simulink model "LSM_4p6U10_v01_06022022_NEW_ECC_2019a"  (R2019a)
settings: Solver=FixedStepAuto  StartTime=0.0  StopTime=Inf  FixedStep=Ts_lowspeed  RelTol=1e-3  EnableMultiTasking=on
PostLoadFcn:
  | , if any(exist('dsrtsu_mdlpostloadfcn', 'file') == [2, 3, 6]), try dsrtsu_mdlpostloadfcn('Execute', bdroot); catch fprintf('Error in PostLoadFcn (dsrtsu_mdlpostloadfcn) for model "%s":\n %s\n', bdroot, lasterr); end, end,
values from neighbouring files (symbols this model uses):
  Ts_lowspeed = 0.05    [Parameters_4p6U10.m]
undefined symbols (not defined in the file or in its folder): Down, GPTRIP1SEL, GPTRIP2SEL, TZ1, TZ2, Up
libraries: simulink x91, simulink_extras x25, c2802xlib x12, c2837xDlib x8, c280xlib x8
(part 1 of 2)
PreSaveFcn:
  | , if any(exist('dsmpb_private', 'file') == [2, 3, 6]), try, dsmpb_private('dsmpb_mdlclblib', 'PreSave', bdroot); catch, disp(lasterr); end, end,
CloseFcn:
  | , if any(exist('dsmpb_private', 'file') == [2, 3, 6]), try, dsmpb_private('dsmpb_mdlclblib', 'Close', bdroot); catch, disp(lasterr); end, end,
settings Model: DSRTSU_INTERNAL_RTI_VER=500  DSRTSU_INTERNAL_RTI_TYPE=rti1007  DSRTSU_INTERNAL_RTIFPGA=90  DSMPB_DATASERVER_ModelPortLibVersion1=8  DSMPB_DATASERVER_DataServerVersion1=6  DSMPB_DATASERVER_DataServerStreamVersion1=3  SimulationMode=external  ExtModeTrigDuration=8  Creator=Christos  LastModifiedBy=ThermoLift
settings DataIOCC: ReturnWorkspaceOutputs=off
settings OptimizationCC: BlockReduction=off  ConditionallyExecuteInputs=off  DefaultUnderspecifiedDataType=single  EnhancedBackFolding=on  PassReuseOutputArgsAs=Individual arguments  MaxStackSize=512  OptimizeBlockOrder=speed
settings DebuggingCC: AlgebraicLoopMsg=none  ArtificialAlgebraicLoopMsg=none  ParameterPrecisionLossMsg=none  ParameterTunabilityLossMsg=error  SFUnexpectedBacktrackingDiag=warning  SFNoUnconditionalDefaultTransitionDiag=warning  SFExecutionAtInitializationDiag=none  ArithmeticOperatorsInVariantConditions=warning
settings HardwareCC: ProdBitPerChar=16  ProdBitPerInt=16  ProdBitPerPointer=32  ProdBitPerSizeT=32  ProdBitPerPtrDiffT=32  ProdLargestAtomicInteger=Integer  ProdLargestAtomicFloat=None  ProdWordSize=16  ProdLongLongMode=on  ProdHWDeviceType=Texas Instruments->C2000  TargetIntDivRoundTo=Zero  TargetEndianess=BigEndian  TargetHWDeviceType=Custom Processor->Custom
settings SFSimCC: SimUseLocalCustomCode=off  MATLABDynamicMemAlloc=off
settings RTWCC: SystemTargetFile=ert.tlc  HardwareBoard=TI Delfino F28379D LaunchPad  TLCOptions=-aInlineSetEventsForThisBaseRateFcn=TLC_FALSE -aSuppressMultiTaskScheduler=TLC_FALSE -aRateBasedStepFcn=1  TemplateMakefile=ert_default_tmf  GenerateReport=on  RTWUseLocalCustomCode=off  RTWUseSimCustomCode=on  Toolchain=Texas Instruments Code Composer Studio (C2000)  IncludeHyperlinkInReport=on  LaunchReport=on  GenerateTraceInfo=on  GenerateTraceReport=on  GenerateTraceReportSl=on  GenerateTraceReportSf=on  GenerateTraceReportEml=on
settings CodeAppCC: ForceParamTrailComments=on  IgnoreCustomStorageClasses=off  OperatorAnnotations=on  SimulinkDataObjDesc=on  SFDataObjDesc=on  InsertBlockDesc=on  StateflowObjectComments=on
settings ERTTargetCC: CodeReplacementLibrary=TI C28x  SupportContinuousTime=on
settings ConfigComp: CovMetricSettings=dw  CovSaveCumulativeToWorkspaceVar=on  CovSaveSingleToWorkspaceVar=on  CovExternalEMLEnable=off
settings SimscapeCC: SimscapeNormalizeSystem=off

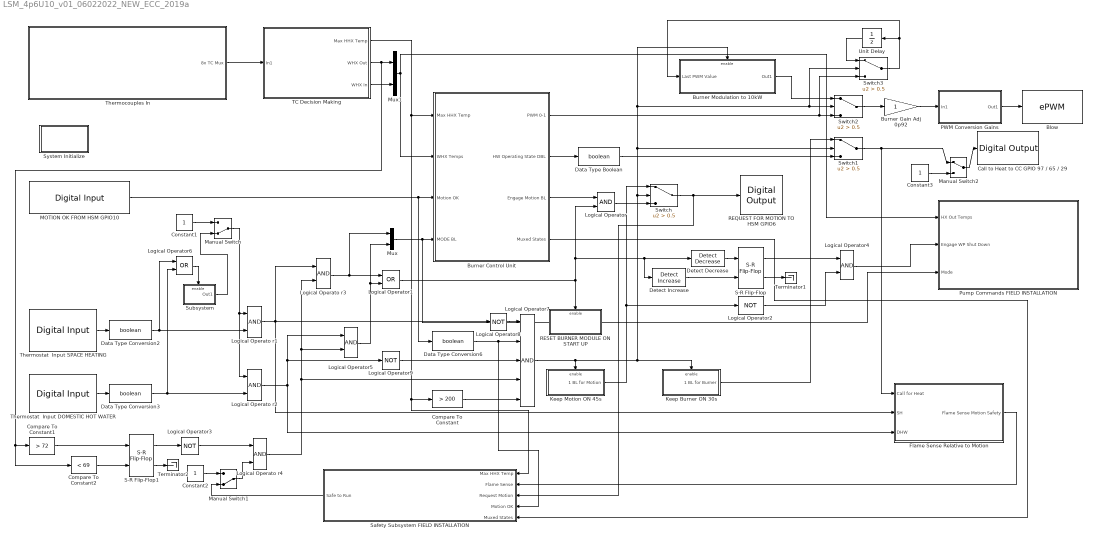
== system LSM_4p6U10_v01_06022022_NEW_ECC_2019a ==
  Blow : c2802xlib/ePWM  useModule=ePWM3  ePWMxLINKTBPRD=Not Linked  periodUnits=Clock cycles  timerSource=Specify via dialog  timerPeriod_clk=16000  timerPeriod_sec=0.0001  tbshadow=Counter equals to zero  countingMode=Up-Down  phaseActiveEnable=Disable  phaseDirection=Count down after sync  phaseActive=0  synchronizationEnable=off  dcaevt1Sync=off  dcbevt1Sync=off  synchronizationOption=Disable  clockPrescale=1  HSclockPrescale=1  enswap=off  ePWMxAStatus=off  ePWMxAactionLogic1=Set  ePWMxAactionLogic2=Clear  ePWMxAactionLogic3=Clear  ePWMxAactionLogic4=Set  ePWMxAactionLogic5=Do nothing  ePWMxAactionLogic6=Do nothing  ePWMxALoadMode=Load on counter equals to zero (CTR=Zero)  ePWMxACSFenable=off  ePWMxACSFvalue=Forcing disable  ePWMxASFreload=Zero  ePWMxBStatus=on  ePWMxBactionLogic1=Set  ePWMxBactionLogic2=Clear  ePWMxBactionLogic3=Clear  ePWMxBactionLogic4=Set  ePWMxBactionLogic5=Do nothing  ePWMxBactionLogic6=Do nothing  ePWMxBLoadMode=Load on counter equals to zero (CTR=Zero)  ePWMxBCSFenable=off  ePWMxBCSFvalue=Forcing disable  ePWMxBSFreload=Zero  ePWNxBOutWay=off  ePWMxLINKCMPA=Not Linked  CMPAUnits=Clock cycles  CMPASource=Input port  CMPAValue_per=0  CMPAValue_clk=32000  enCMPAshadow=Counter equals to zero  ePWMxLINKCMPB=Not Linked  CMPBUnits=Clock cycles  CMPBSource=Specify via dialog  CMPBValue_per=50  CMPBValue_clk=32000  enCMPBshadow=Counter equals to zero  ePWMxLINKCMPC=Not Linked  CMPCUnits=Clock cycles  CMPCSource=Specify via dialog  CMPCValue_per=50  CMPCValue_clk=032000  enCMPCshadow=Counter equals to zero  ePWMxLINKCMPD=Not Linked  CMPDUnits=Clock cycles  CMPDSource=Specify via dialog  CMPDValue_per=50  CMPDValue_clk=32000  enCMPDshadow=Counter equals to zero  enableDBePWMxA=off  enableDBePWMxB=off  enhalfcycle=off  DBpolarity=Active high (AH)  DBedgeDelay=Positive  DBSource_ePWMxA=ePWMxA  DBSource_ePWMxB=ePWMxA  DBperiodSource=Specify via dialog  REDperiod=0  FEDperiod=0  adcstartModuleA=off  adcrequestEventA=First event  adcstartEventA=Digital Compare Module A Event 1 start of conversion (DCAEVT1.soc)  adcstartEventA_type2=Digital Compare Module A Event 1 start of conversion (DCAEVT1.soc)  adcstartModuleB=off  adcrequestEventB=First event  adcstartEventB=Counter equals to zero (CTR=Zero)  adcstartEventB_type2=Counter equals to zero (CTR=Zero)  intEn=off  intPrd=First event  intSel=Counter equals to zero (CTR=Zero)  intSel_type2=Counter equals to zero (CTR=Zero)  hrpe=off  enHRPWM=off  HRPWM_LoadMode=Counter equals to period (CTR=PRD)  HRPWM_CTLMode=Duty or Period control mode  HRPWM_EDGMode=Both edge  hrpeb=off  enHRPWMB=off  HRPWM_LoadModeB=Counter equals to zero (CTR=ZERO)  HRPWM_CTLModeB=Duty or Period control mode  HRPWM_EDGModeB=Both edge  enSFO=on  enautoconv=on  chopperEnable=off  chopperFrequency=1  chopperFirstwidth=1  chopperDuty=12.5%  tripZonesource=Specify via dialog  tzselOSHT1=off  tzselOSHT2=off  tzselOSHT3=off  tzselOSHDCAEV1=off  tzselOSHDCBEV1=off  tzselCBC1=off  tzselCBC2=off  tzselCBC3=off  tzselCBCDCAEV2=off  tzselCBCDCBEV2=off  tzselOSHT4=off  tzselOSHT5=off  tzselOSHT6=off  tzselCBC4=off  tzselCBC5=off  tzselCBC6=off  enTzOstIntr=off  enTzCbcIntr=off  enTzDCAEVT1Intr=off  enTzDCAEVT2Intr=off  enTzDCBEVT1Intr=off  enTzDCBEVT2Intr=off  ePWMxAforced=No action  ePWMxBforced=No action  DCAEVT1forced=No action  DCBEVT1forced=No action  DCAEVT2forced=No action  DCBEVT2forced=No action  dcah=Trip Zone 1 input (TZ1)  dcal=Trip Zone 2 input (TZ2)  dcbh=Trip Zone 1 input (TZ1)  dcbl=Trip Zone 2 input (TZ2)  dcah_type2=GPTRIP1SEL/(TZ1)  dcal_type2=GPTRIP2SEL/(TZ2)  dcbh_type2=GPTRIP1SEL/(TZ1)  dcbl_type2=GPTRIP2SEL/(TZ2)  gendcaevt1=Event disabled  gendcaevt2=Event disabled  gendcbevt1=Event disabled  gendcbevt2=Event disabled  dcaevt1src=DCAEVT1 with sync  dcaevt2src=DCAEVT2 with sync  dcbevt1src=DCBEVT1 with sync  dcbevt2src=DCBEVT2 with sync  pulsesel=Counter equals to zero (CTR=Zero)  blankinv=off  blankoffset=0  blankwidth=0  evsrcsel=Filtered version of DCAEVT1 (DCAEVT1FILT)  encape=off  PwmType=C2000_Type4
  Burner Gain Adj 0p92 : Gain
  Burner Control Unit : Subsystem
  Burner Modulation to 10kW : Subsystem
  Call to Heat to CC GPIO 97 / 65 / 29 : c2837xDlib/Digital Output  GPIO_Number=GPIO0~GPIO7  GPIO_Bit0=off  GPIO_BIT0_Toggle=off  GPIO_Bit1=off  GPIO_BIT1_Toggle=off  GPIO_Bit2=off  GPIO_BIT2_Toggle=off  GPIO_Bit3=on  GPIO_BIT3_Toggle=off  GPIO_Bit4=off  GPIO_BIT4_Toggle=off  GPIO_Bit5=off  GPIO_BIT5_Toggle=off  GPIO_Bit6=off  GPIO_BIT6_Toggle=off  GPIO_Bit7=off  GPIO_BIT7_Toggle=off
      settings: SourceProductBaseCode=TIC2000
  Compare To Constant : simulink/Logic and Bit Operations/Compare To Constant  relop=>  const=200  OutDataTypeStr=boolean
  Compare To Constant1 : simulink/Logic and Bit Operations/Compare To Constant  relop=>  const=72  OutDataTypeStr=boolean
  Compare To Constant2 : simulink/Logic and Bit Operations/Compare To Constant  relop=<  const=69  OutDataTypeStr=boolean
  Constant1 : Constant  OutDataTypeStr=boolean
  Constant2 : Constant  OutDataTypeStr=boolean
  Constant3 : Constant  OutDataTypeStr=boolean
  Data Type Boolean : DataTypeConversion  OutDataTypeStr=boolean
  Data Type Conversion2 : DataTypeConversion  OutDataTypeStr=boolean
  Data Type Conversion3 : DataTypeConversion  OutDataTypeStr=boolean
  Data Type Conversion6 : DataTypeConversion  OutDataTypeStr=boolean
  Detect Decrease : simulink/Logic and Bit Operations/Detect Decrease  vinit=0.0  OutDataTypeStr=boolean
  Detect Increase : simulink/Logic and Bit Operations/Detect Increase  vinit=0.0  OutDataTypeStr=boolean
  Flame Sense Relative to Motion : Subsystem
  Keep Burner ON 30s : Subsystem
  Keep Motion ON 45s : Subsystem
  Logical Operato r{1..4} (4 alike) : Logic  AllPortsSameDT=off  OutDataTypeStr=boolean
  Logical Operator : Logic  AllPortsSameDT=off  OutDataTypeStr=boolean
  Logical Operator1 : Logic  Operator=OR  AllPortsSameDT=off  OutDataTypeStr=boolean
  Logical Operator{2..3,8..9} (4 alike) : Logic  Operator=NOT  AllPortsSameDT=off  OutDataTypeStr=boolean
  Logical Operator4 : Logic  AllPortsSameDT=off  OutDataTypeStr=boolean
  Logical Operator5 : Logic  AllPortsSameDT=off  OutDataTypeStr=boolean
  Logical Operator6 : Logic  Operator=OR  AllPortsSameDT=off  OutDataTypeStr=boolean
  Logical Operator7 : Logic  Inputs=5  AllPortsSameDT=off  OutDataTypeStr=boolean
  MOTION OK FROM HSM GPIO10 : c2837xDlib/Digital Input  GPIO_Number=GPIO8~GPIO15  GPIO_Bit0=off  GPIO_Bit1=off  GPIO_Bit2=on  GPIO_Bit3=off  GPIO_Bit4=off  GPIO_Bit5=off  GPIO_Bit6=off  GPIO_Bit7=off  sampleTime=Ts_lowspeed  dataType=boolean  GPIO_Bit0_Qualification=Sync to SYSCLKOUT  GPIO_Bit1_Qualification=Sync to SYSCLKOUT  GPIO_Bit2_Qualification=Sync to SYSCLKOUT  GPIO_Bit3_Qualification=Sync to SYSCLKOUT  GPIO_Bit4_Qualification=Sync to SYSCLKOUT  GPIO_Bit5_Qualification=Sync to SYSCLKOUT  GPIO_Bit6_Qualification=Sync to SYSCLKOUT  GPIO_Bit7_Qualification=Sync to SYSCLKOUT  Qualification_Period=-1
      settings: SourceProductBaseCode=TIC2000
  Manual Switch : ManualSwitch  CurrentSetting=0
  Manual Switch1 : ManualSwitch  CurrentSetting=0
  Manual Switch2 : ManualSwitch
  Mux : Mux  Inputs=2
  Mux1 : Mux  Inputs=2
  PWM Conversion Gains : Subsystem
  Pump Commands FIELD INSTALLATION : Subsystem
  REQUEST FOR MOTION TO HSM GPIO6 : c2837xDlib/Digital Output  GPIO_Number=GPIO0~GPIO7  GPIO_Bit0=off  GPIO_BIT0_Toggle=off  GPIO_Bit1=off  GPIO_BIT1_Toggle=off  GPIO_Bit2=off  GPIO_BIT2_Toggle=off  GPIO_Bit3=off  GPIO_BIT3_Toggle=off  GPIO_Bit4=off  GPIO_BIT4_Toggle=off  GPIO_Bit5=off  GPIO_BIT5_Toggle=off  GPIO_Bit6=on  GPIO_BIT6_Toggle=off  GPIO_Bit7=off  GPIO_BIT7_Toggle=off
      settings: SourceProductBaseCode=TIC2000
  RESET BURNER MODULE ON START UP : Subsystem
  S-R Flip-Flop : simulink_extras/Flip Flops/S-R Flip-Flop  initial_condition=0
  S-R Flip-Flop1 : simulink_extras/Flip Flops/S-R Flip-Flop  initial_condition=0
  Safety Subsystem FIELD INSTALLATION : Subsystem
  Subsystem : Subsystem
  Switch{,1..3} (4 alike) : Switch  Criteria=u2 > Threshold  Threshold=0.5
  System Initialize : Subsystem  mask(System Initialize){ShowInLibBrowser=0}
      mask prompts: ShowInLibBrowser "Simulink:masks:CustCodeMaskParam1_MP"
      settings: CopyFcn=cccopyfcn(gcb)  OpenFcn=ccopenfcn('System Initialize Function')
      mask Help: eval('feval(''rtwprivate'',''rtwhelpview'',''rtw_sys_initialize_block'')');
      mask Display: disp('System\nInitialize');
  TC Decision Making : Subsystem
  Terminator1 : Terminator
  Terminator2 : Terminator
  Thermocouples In : Subsystem
  Thermostat  Input DOMESTIC HOT WATER : c2837xDlib/Digital Input  GPIO_Number=GPIO16~GPIO23  GPIO_Bit0=off  GPIO_Bit1=off  GPIO_Bit2=on  GPIO_Bit3=off  GPIO_Bit4=off  GPIO_Bit5=off  GPIO_Bit6=off  GPIO_Bit7=off  sampleTime=Ts_lowspeed  dataType=boolean  GPIO_Bit0_Qualification=Sync to SYSCLKOUT  GPIO_Bit1_Qualification=Sync to SYSCLKOUT  GPIO_Bit2_Qualification=Sync to SYSCLKOUT  GPIO_Bit3_Qualification=Sync to SYSCLKOUT  GPIO_Bit4_Qualification=Sync to SYSCLKOUT  GPIO_Bit5_Qualification=Sync to SYSCLKOUT  GPIO_Bit6_Qualification=Sync to SYSCLKOUT  GPIO_Bit7_Qualification=Sync to SYSCLKOUT  Qualification_Period=-1
      settings: SourceProductBaseCode=TIC2000
  Thermostat  Input SPACE HEATING : c2837xDlib/Digital Input  GPIO_Number=GPIO32~GPIO39  GPIO_Bit0=on  GPIO_Bit1=off  GPIO_Bit2=off  GPIO_Bit3=off  GPIO_Bit4=off  GPIO_Bit5=off  GPIO_Bit6=off  GPIO_Bit7=off  sampleTime=Ts_lowspeed  dataType=boolean  GPIO_Bit0_Qualification=Sync to SYSCLKOUT  GPIO_Bit1_Qualification=Sync to SYSCLKOUT  GPIO_Bit2_Qualification=Sync to SYSCLKOUT  GPIO_Bit3_Qualification=Sync to SYSCLKOUT  GPIO_Bit4_Qualification=Sync to SYSCLKOUT  GPIO_Bit5_Qualification=Sync to SYSCLKOUT  GPIO_Bit6_Qualification=Sync to SYSCLKOUT  GPIO_Bit7_Qualification=Sync to SYSCLKOUT  Qualification_Period=-1
      settings: SourceProductBaseCode=TIC2000
  Unit Delay : UnitDelay  SampleTime=-1  HasFrameUpgradeWarning=on
  wires:
  Logical Operator/1 -> Switch/3
  Mux/1 -> Pump Commands FIELD INSTALLATION/3(Mode), Burner Control Unit/4(MODE BL)
  MOTION OK FROM HSM GPIO10/1 -> Burner Control Unit/3(Motion OK), Data Type Conversion6/1
  Logical Operato r2/1 -> Flame Sense Relative to Motion/3(DHW), Logical Operator5/1, Logical Operator9/1
  Logical Operato r1/1 -> Flame Sense Relative to Motion/2(SH), Logical Operator8/1, Logical Operato r3/1
  Thermostat  Input SPACE HEATING/1 -> Data Type Conversion2/1
  Burner Control Unit/3(Engage Motion BL) -> Logical Operator/1
  Thermostat  Input DOMESTIC HOT WATER/1 -> Data Type Conversion3/1
  Data Type Boolean/1 -> Switch1/3
  Logical Operato r3/1 -> Mux/1, Logical Operator1/1
  Logical Operator1/1 -> RESET BURNER MODULE ON START UP/Enable, Logical Operator/2, Detect Increase/1, Detect Decrease/1
  Logical Operator5/1 -> Mux/2, Logical Operator1/2
  Burner Control Unit/2(HW Operating State DBL) -> Data Type Boolean/1
  Data Type Conversion6/1 -> Safety Subsystem FIELD INSTALLATION/4(Motion OK), Logical Operator7/2
  Logical Operator8/1 -> Logical Operator7/1
  Logical Operator9/1 -> Logical Operator7/3
  Logical Operator7/1 -> Burner Modulation to 10kW/Enable, Switch3/2, Switch2/2, Switch1/2, Switch/2, Keep Burner ON 30s/Enable, Keep Motion ON 45s/Enable
  Keep Motion ON 45s/1(1 BL for Motion) -> Logical Operator2/1, Switch/1
  Keep Burner ON 30s/1(1 BL for Burner) -> Switch1/1
  Switch1/1 -> Flame Sense Relative to Motion/1(Call for Heat), Manual Switch2/1
  Logical Operato r4/1 -> Logical Operato r3/2, Logical Operator5/2, Logical Operator7/4
  Flame Sense Relative to Motion/1(Flame Sense Motion Safety) -> Safety Subsystem FIELD INSTALLATION/2(Flame Sense)
  Switch2/1 -> Burner Gain Adj 0p92/1
  PWM Conversion Gains/1(Out1) -> Blow/1
  Burner Control Unit/1(PWM 0-1) -> Switch3/3, Switch2/3
  Burner Modulation to 10kW/1(Out1) -> Switch2/1
  Detect Decrease/1 -> S-R Flip-Flop/1
  Detect Increase/1 -> S-R Flip-Flop/2
  S-R Flip-Flop/2 -> Terminator1/1
  S-R Flip-Flop/1 -> Logical Operator4/1
  Logical Operator2/1 -> Logical Operator4/2
  Logical Operator4/1 -> Pump Commands FIELD INSTALLATION/2(Engage WP Shut Down)
  Switch3/1 -> Burner Modulation to 10kW/1(Last PWM Value), Unit Delay/1
  Unit Delay/1 -> Switch3/1
  Thermocouples In/1(8x TC Mux) -> TC Decision Making/1(In1)
  TC Decision Making/2(WHX Out) -> Compare To Constant2/1, Compare To Constant1/1, Mux1/1
  TC Decision Making/1(Max HHX Temp) -> Burner Control Unit/1(Max HHX Temp), Safety Subsystem FIELD INSTALLATION/1(Max HHX Temp), Compare To Constant/1
  TC Decision Making/3(WHX In) -> Mux1/2
  Mux1/1 -> Burner Control Unit/2(WHX Temps), Pump Commands FIELD INSTALLATION/1(HX Out Temps)
  Burner Gain Adj 0p92/1 -> PWM Conversion Gains/1(In1)
  Logical Operator6/1 -> Subsystem/Enable
  Manual Switch/1 -> Logical Operato r2/1, Logical Operato r1/1
  Data Type Conversion2/1 -> Logical Operator6/1, Logical Operato r1/2
  Data Type Conversion3/1 -> Logical Operator6/2, Logical Operato r2/2
  Subsystem/1(Out1) -> Manual Switch/2
  Constant1/1 -> Manual Switch/1
  Compare To Constant/1 -> Logical Operator7/5
  Burner Control Unit/4(Muxed States) -> Safety Subsystem FIELD INSTALLATION/5(Muxed States)
  Compare To Constant1/1 -> S-R Flip-Flop1/1
  Compare To Constant2/1 -> S-R Flip-Flop1/2
  S-R Flip-Flop1/1 -> Logical Operator3/1
  S-R Flip-Flop1/2 -> Terminator2/1
  Logical Operator3/1 -> Logical Operato r4/1
  Safety Subsystem FIELD INSTALLATION/1(Safe to Run) -> Manual Switch1/2
  Constant2/1 -> Manual Switch1/1
  Manual Switch1/1 -> Logical Operato r4/2
  Switch/1 -> REQUEST FOR MOTION TO HSM GPIO6/1, Safety Subsystem FIELD INSTALLATION/3(Request Motion)
  Constant3/1 -> Manual Switch2/2
  Manual Switch2/1 -> Call to Heat to CC GPIO 97 / 65 / 29/1

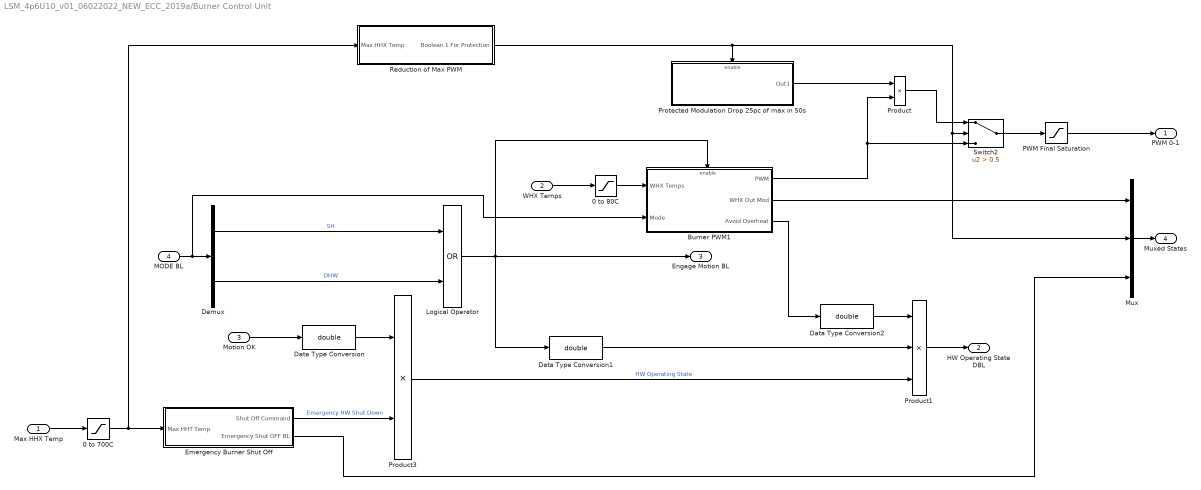
== system LSM_4p6U10_v01_06022022_NEW_ECC_2019a/Burner Control Unit ==
  Max HHX Temp : Inport
  WHX Temps : Inport  Port=2
  Motion OK : Inport  Port=3
  MODE BL : Inport  Port=4
  0 to 700C : Saturate  UpperLimit=705  LowerLimit=0
  0 to 80C : Saturate  UpperLimit=80  LowerLimit=0
  Burner PWM1 : Subsystem
  Data Type Conversion : DataTypeConversion  OutDataTypeStr=double
  Data Type Conversion1 : DataTypeConversion  OutDataTypeStr=double
  Data Type Conversion2 : DataTypeConversion  OutDataTypeStr=double
  Demux : Demux  Outputs=2
  Emergency Burner Shut Off : Subsystem
  Logical Operator : Logic  Operator=OR  AllPortsSameDT=off  OutDataTypeStr=boolean
  Mux : Mux  Inputs=3
  "PWM Final Saturation " : Saturate  UpperLimit=0.41  LowerLimit=0.2
  Product : Product
  Product1 : Product  Inputs=3
  Product3 : Product
  Protected Modulation Drop 25pc of max in 50s : Subsystem
  Reduction of Max PWM : Subsystem
  Switch2 : Switch  Criteria=u2 > Threshold  Threshold=0.5
  PWM 0-1 : Outport  VectorParamsAs1DForOutWhenUnconnected=on
  HW Operating State DBL : Outport  Port=2  VectorParamsAs1DForOutWhenUnconnected=on
  Engage Motion BL : Outport  Port=3  VectorParamsAs1DForOutWhenUnconnected=on
  Muxed States : Outport  Port=4  VectorParamsAs1DForOutWhenUnconnected=on
  wires:
  Max HHX Temp/1 -> 0 to 700C/1
  Emergency Burner Shut Off/1(Shut Off Command) -> Product3/2  "Emergency HW Shut Down"
  Data Type Conversion/1 -> Product3/1
  Motion OK/1 -> Data Type Conversion/1
  Product3/1 -> Product1/3  "HW Operating State"
  Product/1 -> Switch2/1
  Reduction of Max PWM/1(Boolean 1 For Protection) -> Mux/2, Switch2/2, Protected Modulation Drop 25pc of max in 50s/Enable
  0 to 700C/1 -> Reduction of Max PWM/1(Max HHX Temp), Emergency Burner Shut Off/1(Max HHT Temp)
  MODE BL/1 -> Burner PWM1/2(Mode), Demux/1
  Demux/1 -> Logical Operator/1  "SH"
  Demux/2 -> Logical Operator/2  "DHW"
  WHX Temps/1 -> 0 to 80C/1
  Product1/1 -> HW Operating State DBL/1
  Data Type Conversion1/1 -> Product1/2
  Protected Modulation Drop 25pc of max in 50s/1(Out1) -> Product/1
  Burner PWM1/1(PWM) -> Product/2, Switch2/3
  Switch2/1 -> "PWM Final Saturation "/1
  "PWM Final Saturation "/1 -> PWM 0-1/1
  Emergency Burner Shut Off/2(Emergency Shut OFF BL) -> Mux/3
  Burner PWM1/2(WHX Out Mod) -> Mux/1
  Mux/1 -> Muxed States/1
  Burner PWM1/3(Avoid Overheat) -> Data Type Conversion2/1
  Data Type Conversion2/1 -> Product1/1
  Logical Operator/1 -> Engage Motion BL/1, Burner PWM1/Enable, Data Type Conversion1/1
  0 to 80C/1 -> Burner PWM1/1(WHX Temps)

== system LSM_4p6U10_v01_06022022_NEW_ECC_2019a/Burner Modulation to 10kW ==
  Last PWM Value : Inport
  Enable : EnablePort  StatesWhenEnabling=reset
  Constant : Constant
  Gain : Gain  Gain=-0.0030
  Integrator : Integrator  LimitOutput=on  UpperSaturationLimit=300  LowerSaturationLimit=0
  Limit Saturation : Saturate  UpperLimit=1  LowerLimit=0.7
  PWM Limits 41 to 24p6 : Saturate  UpperLimit=0.41  LowerLimit=0.246
  Product : Product
  Sum : Sum  Inputs=|++
  Unit : Constant
  Out1 : Outport
  wires:
  Constant/1 -> Integrator/1
  Integrator/1 -> Gain/1
  Gain/1 -> Sum/1
  Unit/1 -> Sum/2
  Sum/1 -> Limit Saturation/1
  Limit Saturation/1 -> Product/1
  Product/1 -> PWM Limits 41 to 24p6/1
  Last PWM Value/1 -> Product/2
  PWM Limits 41 to 24p6/1 -> Out1/1

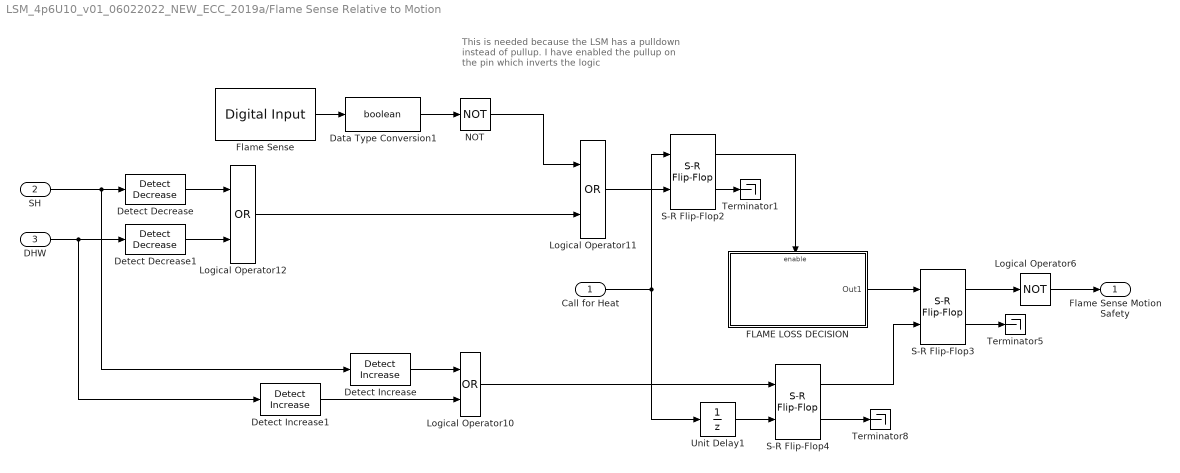
== system LSM_4p6U10_v01_06022022_NEW_ECC_2019a/Flame Sense Relative to Motion ==
  note: This is needed because the LSM has a pulldown instead of pullup. I have enabled the pullup on the pin which inverts the logic
  Call for Heat : Inport
  SH : Inport  Port=2
  DHW : Inport  Port=3
  Data Type Conversion1 : DataTypeConversion  OutDataTypeStr=boolean
  Detect Decrease : simulink/Logic and Bit Operations/Detect Decrease  vinit=0.0  OutDataTypeStr=boolean
  Detect Decrease1 : simulink/Logic and Bit Operations/Detect Decrease  vinit=0.0  OutDataTypeStr=boolean
  Detect Increase : simulink/Logic and Bit Operations/Detect Increase  vinit=0.0  OutDataTypeStr=boolean
  Detect Increase1 : simulink/Logic and Bit Operations/Detect Increase  vinit=0.0  OutDataTypeStr=boolean
  FLAME LOSS DECISION : Subsystem
  Flame Sense : c2837xDlib/Digital Input  GPIO_Number=GPIO64~GPIO71  GPIO_Bit0=off  GPIO_Bit1=on  GPIO_Bit2=off  GPIO_Bit3=off  GPIO_Bit4=off  GPIO_Bit5=off  GPIO_Bit6=off  GPIO_Bit7=off  sampleTime=Ts_lowspeed  dataType=boolean  GPIO_Bit0_Qualification=Sync to SYSCLKOUT  GPIO_Bit1_Qualification=Sync to SYSCLKOUT  GPIO_Bit2_Qualification=Sync to SYSCLKOUT  GPIO_Bit3_Qualification=Sync to SYSCLKOUT  GPIO_Bit4_Qualification=Sync to SYSCLKOUT  GPIO_Bit5_Qualification=Sync to SYSCLKOUT  GPIO_Bit6_Qualification=Sync to SYSCLKOUT  GPIO_Bit7_Qualification=Sync to SYSCLKOUT  Qualification_Period=-1
      settings: SourceProductBaseCode=TIC2000
  Logical Operator10 : Logic  Operator=OR  AllPortsSameDT=off  OutDataTypeStr=boolean
  Logical Operator11 : Logic  Operator=OR  AllPortsSameDT=off  OutDataTypeStr=boolean
  Logical Operator12 : Logic  Operator=OR  AllPortsSameDT=off  OutDataTypeStr=boolean
  Logical Operator6 : Logic  Operator=NOT  AllPortsSameDT=off  OutDataTypeStr=boolean
  NOT : Logic  Operator=NOT  IconShape=distinctive  AllPortsSameDT=off  OutDataTypeStr=boolean
  S-R Flip-Flop2 : simulink_extras/Flip Flops/S-R Flip-Flop  initial_condition=0
  S-R Flip-Flop3 : simulink_extras/Flip Flops/S-R Flip-Flop  initial_condition=0
  S-R Flip-Flop4 : simulink_extras/Flip Flops/S-R Flip-Flop  initial_condition=0
  Terminator1 : Terminator
  Terminator5 : Terminator
  Terminator8 : Terminator
  Unit Delay1 : UnitDelay  SampleTime=-1  HasFrameUpgradeWarning=on
  Flame Sense Motion Safety : Outport
  wires:
  S-R Flip-Flop2/2 -> Terminator1/1
  S-R Flip-Flop3/1 -> Logical Operator6/1
  DHW/1 -> Detect Decrease1/1, Detect Increase1/1
  SH/1 -> Detect Increase/1, Detect Decrease/1
  S-R Flip-Flop2/1 -> FLAME LOSS DECISION/Enable
  Detect Decrease1/1 -> Logical Operator12/2
  Call for Heat/1 -> S-R Flip-Flop2/1, Unit Delay1/1
  S-R Flip-Flop4/1 -> S-R Flip-Flop3/2
  Detect Decrease/1 -> Logical Operator12/1
  Detect Increase/1 -> Logical Operator10/1
  S-R Flip-Flop3/2 -> Terminator5/1
  Flame Sense/1 -> Data Type Conversion1/1
  Logical Operator11/1 -> S-R Flip-Flop2/2
  S-R Flip-Flop4/2 -> Terminator8/1
  FLAME LOSS DECISION/1(Out1) -> S-R Flip-Flop3/1
  Detect Increase1/1 -> Logical Operator10/2
  Logical Operator12/1 -> Logical Operator11/2
  Unit Delay1/1 -> S-R Flip-Flop4/2
  Logical Operator10/1 -> S-R Flip-Flop4/1
  Logical Operator6/1 -> Flame Sense Motion Safety/1
  Data Type Conversion1/1 -> NOT/1
  NOT/1 -> Logical Operator11/1

== system LSM_4p6U10_v01_06022022_NEW_ECC_2019a/Keep Burner ON 30s ==
  Enable : EnablePort  StatesWhenEnabling=reset
  0 to 151 : Integrator  LimitOutput=on  UpperSaturationLimit=151  LowerSaturationLimit=0
  Compare To Constant : simulink/Logic and Bit Operations/Compare To Constant  relop=<  const=30  OutDataTypeStr=boolean
  Constant : Constant
  1 BL for Burner : Outport
  wires:
  Compare To Constant/1 -> 1 BL for Burner/1
  0 to 151/1 -> Compare To Constant/1
  Constant/1 -> 0 to 151/1

== system LSM_4p6U10_v01_06022022_NEW_ECC_2019a/Keep Motion ON 45s ==
  Enable : EnablePort  StatesWhenEnabling=reset
  0 to 151 : Integrator  LimitOutput=on  UpperSaturationLimit=151  LowerSaturationLimit=0
  Compare To Constant : simulink/Logic and Bit Operations/Compare To Constant  relop=<  const=45  OutDataTypeStr=boolean
  Constant : Constant
  1 BL for Motion : Outport
  wires:
  Constant/1 -> 0 to 151/1
  0 to 151/1 -> Compare To Constant/1
  Compare To Constant/1 -> 1 BL for Motion/1

== system LSM_4p6U10_v01_06022022_NEW_ECC_2019a/PWM Conversion Gains ==
  In1 : Inport
  Cast To Double3 : DataTypeConversion  OutDataTypeStr=uint16
  Ceil3 : Rounding  Operator=ceil
  Gain : Gain  Gain=16000
  Out1 : Outport
  wires:
  Ceil3/1 -> Cast To Double3/1
  Gain/1 -> Ceil3/1
  In1/1 -> Gain/1
  Cast To Double3/1 -> Out1/1

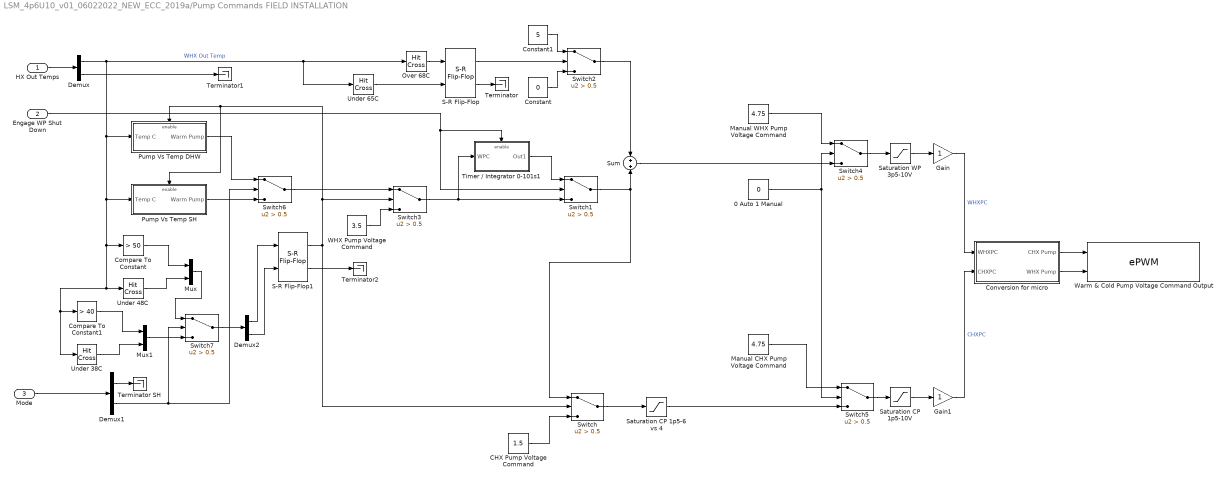
== system LSM_4p6U10_v01_06022022_NEW_ECC_2019a/Pump Commands FIELD INSTALLATION ==
  HX Out Temps : Inport
  Engage WP Shut Down : Inport  Port=2
  Mode : Inport  Port=3
  0 Auto 1 Manual : Constant  Value=0  OutDataTypeStr=boolean
  CHX Pump Voltage Command : Constant  Value=1.5
  Compare To Constant : simulink/Logic and Bit Operations/Compare To Constant  relop=>  const=50  OutDataTypeStr=boolean
  Compare To Constant1 : simulink/Logic and Bit Operations/Compare To Constant  relop=>  const=40  OutDataTypeStr=boolean
  Constant : Constant  Value=0
  Constant1 : Constant  Value=5
  Conversion for micro : Subsystem
  Demux : Demux  Outputs=2
  Demux1 : Demux  Outputs=2
  Demux2 : Demux  Outputs=2
  Gain : Gain
  Gain1 : Gain
  Manual CHX Pump Voltage Command : Constant  Value=4.75
  Manual WHX Pump Voltage Command : Constant  Value=4.75
  Mux : Mux  Inputs=2
  Mux1 : Mux  Inputs=2
  Over 68C : HitCross  HitCrossingOffset=68  HitCrossingDirection=rising
  Pump Vs Temp DHW : Subsystem
  Pump Vs Temp SH : Subsystem
  S-R Flip-Flop : simulink_extras/Flip Flops/S-R Flip-Flop  initial_condition=0
  S-R Flip-Flop1 : simulink_extras/Flip Flops/S-R Flip-Flop  initial_condition=0
  Saturation CP 1p5-10V : Saturate  UpperLimit=10  LowerLimit=1.5
  Saturation CP 1p5-6 vs 4 : Saturate  UpperLimit=4  LowerLimit=1.5
  Saturation WP 3p5-10V : Saturate  UpperLimit=10  LowerLimit=3.5
  Sum : Sum
  Switch{,1..7} (8 alike) : Switch  Criteria=u2 > Threshold  Threshold=0.5
  Terminator : Terminator
  Terminator SH : Terminator
  Terminator1 : Terminator
  Terminator2 : Terminator
  Timer / Integrator 0-101s1 : Subsystem
  Under 38C : HitCross  HitCrossingOffset=38  HitCrossingDirection=falling
  Under 48C : HitCross  HitCrossingOffset=48  HitCrossingDirection=falling
  Under 65C : HitCross  HitCrossingOffset=65  HitCrossingDirection=falling
  WHX Pump Voltage Command : Constant  Value=3.5
  Warm & Cold Pump Voltage Command Output : c2802xlib/ePWM  useModule=ePWM1  ePWMxLINKTBPRD=Not Linked  periodUnits=Clock cycles  timerSource=Specify via dialog  timerPeriod_clk=1023  timerPeriod_sec=0.0001  tbshadow=Counter equals to zero  countingMode=Up  phaseActiveEnable=Disable  phaseDirection=Count down after sync  phaseActive=0  synchronizationEnable=off  dcaevt1Sync=off  dcbevt1Sync=off  synchronizationOption=Disable  clockPrescale=1  HSclockPrescale=1  enswap=off  ePWMxAStatus=on  ePWMxAactionLogic1=Do nothing  ePWMxAactionLogic2=Set  ePWMxAactionLogic3=Clear  ePWMxAactionLogic4=Set  ePWMxAactionLogic5=Do nothing  ePWMxAactionLogic6=Do nothing  ePWMxALoadMode=Load on counter equals to zero (CTR=Zero)  ePWMxACSFenable=off  ePWMxACSFvalue=Forcing disable  ePWMxASFreload=Zero  ePWMxBStatus=on  ePWMxBactionLogic1=Do nothing  ePWMxBactionLogic2=Set  ePWMxBactionLogic3=Do nothing  ePWMxBactionLogic4=Do nothing  ePWMxBactionLogic5=Clear  ePWMxBactionLogic6=Set  ePWMxBLoadMode=Load on counter equals to zero (CTR=Zero)  ePWMxBCSFenable=off  ePWMxBCSFvalue=Forcing disable  ePWMxBSFreload=Zero  ePWNxBOutWay=off  ePWMxLINKCMPA=Not Linked  CMPAUnits=Clock cycles  CMPASource=Input port  CMPAValue_per=50  CMPAValue_clk=0  enCMPAshadow=Counter equals to zero  ePWMxLINKCMPB=Not Linked  CMPBUnits=Clock cycles  CMPBSource=Input port  CMPBValue_per=50  CMPBValue_clk=0  enCMPBshadow=Counter equals to zero  ePWMxLINKCMPC=Not Linked  CMPCUnits=Clock cycles  CMPCSource=Specify via dialog  CMPCValue_per=50  CMPCValue_clk=0  enCMPCshadow=Counter equals to zero  ePWMxLINKCMPD=Not Linked  CMPDUnits=Clock cycles  CMPDSource=Specify via dialog  CMPDValue_per=50  CMPDValue_clk=0  enCMPDshadow=Counter equals to zero  enableDBePWMxA=off  enableDBePWMxB=off  enhalfcycle=off  DBpolarity=Active high (AH)  DBedgeDelay=Positive  DBSource_ePWMxA=ePWMxA  DBSource_ePWMxB=ePWMxA  DBperiodSource=Specify via dialog  REDperiod=0  FEDperiod=0  adcstartModuleA=off  adcrequestEventA=First event  adcstartEventA=Digital Compare Module A Event 1 start of conversion (DCAEVT1.soc)  adcstartEventA_type2=Digital Compare Module A Event 1 start of conversion (DCAEVT1.soc)  adcstartModuleB=off  adcrequestEventB=First event  adcstartEventB=Counter equals to zero (CTR=Zero)  adcstartEventB_type2=Counter equals to zero (CTR=Zero)  intEn=off  intPrd=First event  intSel=Counter equals to zero (CTR=Zero)  intSel_type2=Counter equals to zero (CTR=Zero)  hrpe=off  enHRPWM=off  HRPWM_LoadMode=Counter equals to period (CTR=PRD)  HRPWM_CTLMode=Duty or Period control mode  HRPWM_EDGMode=Both edge  hrpeb=off  enHRPWMB=off  HRPWM_LoadModeB=Counter equals to zero (CTR=ZERO)  HRPWM_CTLModeB=Duty or Period control mode  HRPWM_EDGModeB=Both edge  enSFO=on  enautoconv=on  chopperEnable=off  chopperFrequency=1  chopperFirstwidth=1  chopperDuty=12.5%  tripZonesource=Specify via dialog  tzselOSHT1=off  tzselOSHT2=off  tzselOSHT3=off  tzselOSHDCAEV1=off  tzselOSHDCBEV1=off  tzselCBC1=off  tzselCBC2=off  tzselCBC3=off  tzselCBCDCAEV2=off  tzselCBCDCBEV2=off  tzselOSHT4=off  tzselOSHT5=off  tzselOSHT6=off  tzselCBC4=off  tzselCBC5=off  tzselCBC6=off  enTzOstIntr=off  enTzCbcIntr=off  enTzDCAEVT1Intr=off  enTzDCAEVT2Intr=off  enTzDCBEVT1Intr=off  enTzDCBEVT2Intr=off  ePWMxAforced=No action  ePWMxBforced=No action  DCAEVT1forced=No action  DCBEVT1forced=No action  DCAEVT2forced=No action  DCBEVT2forced=No action  dcah=Trip Zone 1 input (TZ1)  dcal=Trip Zone 2 input (TZ2)  dcbh=Trip Zone 1 input (TZ1)  dcbl=Trip Zone 2 input (TZ2)  dcah_type2=GPTRIP1SEL/(TZ1)  dcal_type2=GPTRIP2SEL/(TZ2)  dcbh_type2=GPTRIP1SEL/(TZ1)  dcbl_type2=GPTRIP2SEL/(TZ2)  gendcaevt1=Event disabled  gendcaevt2=Event disabled  gendcbevt1=Event disabled  gendcbevt2=Event disabled  dcaevt1src=DCAEVT1 with sync  dcaevt2src=DCAEVT2 with sync  dcbevt1src=DCBEVT1 with sync  dcbevt2src=DCBEVT2 with sync  pulsesel=Counter equals to zero (CTR=Zero)  blankinv=off  blankoffset=0  blankwidth=0  evsrcsel=Filtered version of DCAEVT1 (DCAEVT1FILT)  encape=off  PwmType=C2000_Type4
  wires:
  Conversion for micro/1(CHX Pump) -> Warm & Cold Pump Voltage Command Output/1
  Conversion for micro/2(WHX Pump) -> Warm & Cold Pump Voltage Command Output/2
  Switch1/1 -> Switch/1, Sum/2
  Switch3/1 -> Timer / Integrator 0-101s1/1(WPC), Switch1/3
  Mux1/1 -> Switch7/3
  Under 38C/1 -> Mux1/2
  Under 65C/1 -> S-R Flip-Flop/2
  Demux1/2 -> Switch7/2, Switch6/2
  Pump Vs Temp DHW/1(Warm Pump) -> Switch6/1
  Compare To Constant1/1 -> Mux1/1
  Mux/1 -> Switch7/1
  HX Out Temps/1 -> Demux/1
  Constant1/1 -> Switch2/1
  Switch7/1 -> Demux2/1
  Mode/1 -> Demux1/1
  Gain/1 -> Conversion for micro/1(WHXPC)  "WHXPC"
  Manual WHX Pump Voltage Command/1 -> Switch4/1
  Switch/1 -> Saturation CP 1p5-6 vs 4/1
  Timer / Integrator 0-101s1/1(Out1) -> Switch1/1
  Saturation CP 1p5-6 vs 4/1 -> Switch5/3
  S-R Flip-Flop1/2 -> Terminator2/1
  Under 48C/1 -> Mux/2
  Constant/1 -> Switch2/3
  Demux2/1 -> S-R Flip-Flop1/1
  Pump Vs Temp SH/1(Warm Pump) -> Switch6/3
  Switch4/1 -> Saturation WP 3p5-10V/1
  S-R Flip-Flop1/1 -> Switch/2, Pump Vs Temp SH/Enable, Pump Vs Temp DHW/Enable, Switch3/2
  Demux/2 -> Terminator1/1
  Engage WP Shut Down/1 -> Switch1/2, Timer / Integrator 0-101s1/Enable
  S-R Flip-Flop/2 -> Terminator/1
  Manual CHX Pump Voltage Command/1 -> Switch5/1
  WHX Pump Voltage Command/1 -> Switch3/3
  Switch5/1 -> Saturation CP 1p5-10V/1
  0 Auto 1 Manual/1 -> Switch5/2, Switch4/2
  Switch2/1 -> Sum/1
  Saturation CP 1p5-10V/1 -> Gain1/1
  S-R Flip-Flop/1 -> Switch2/2
  Demux1/1 -> Terminator SH/1
  Over 68C/1 -> S-R Flip-Flop/1
  Gain1/1 -> Conversion for micro/2(CHXPC)  "CHXPC"
  Compare To Constant/1 -> Mux/1
  Demux/1 -> Under 65C/1, Over 68C/1, Pump Vs Temp SH/1(Temp C), Compare To Constant/1, Under 48C/1, Under 38C/1, Compare To Constant1/1, Pump Vs Temp DHW/1(Temp C)  "WHX Out Temp"
  Switch6/1 -> Switch3/1
  Demux2/2 -> S-R Flip-Flop1/2
  CHX Pump Voltage Command/1 -> Switch/3
  Saturation WP 3p5-10V/1 -> Gain/1
  Sum/1 -> Switch4/3

== system LSM_4p6U10_v01_06022022_NEW_ECC_2019a/RESET BURNER MODULE ON START UP ==
  Enable : EnablePort  StatesWhenEnabling=reset
  Compare To Constant : simulink/Logic and Bit Operations/Compare To Constant  relop=<  const=3  OutDataTypeStr=boolean
  Constant : Constant
  Integrator : Integrator  LimitOutput=on  UpperSaturationLimit=5  LowerSaturationLimit=0
  RESET BURNER MODULE : c2837xDlib/Digital Output  GPIO_Number=GPIO0~GPIO7  GPIO_Bit0=off  GPIO_BIT0_Toggle=off  GPIO_Bit1=off  GPIO_BIT1_Toggle=off  GPIO_Bit2=on  GPIO_BIT2_Toggle=off  GPIO_Bit3=off  GPIO_BIT3_Toggle=off  GPIO_Bit4=off  GPIO_BIT4_Toggle=off  GPIO_Bit5=off  GPIO_BIT5_Toggle=off  GPIO_Bit6=off  GPIO_BIT6_Toggle=off  GPIO_Bit7=off  GPIO_BIT7_Toggle=off
      settings: SourceProductBaseCode=TIC2000
  wires:
  Constant/1 -> Integrator/1
  Integrator/1 -> Compare To Constant/1
  Compare To Constant/1 -> RESET BURNER MODULE/1

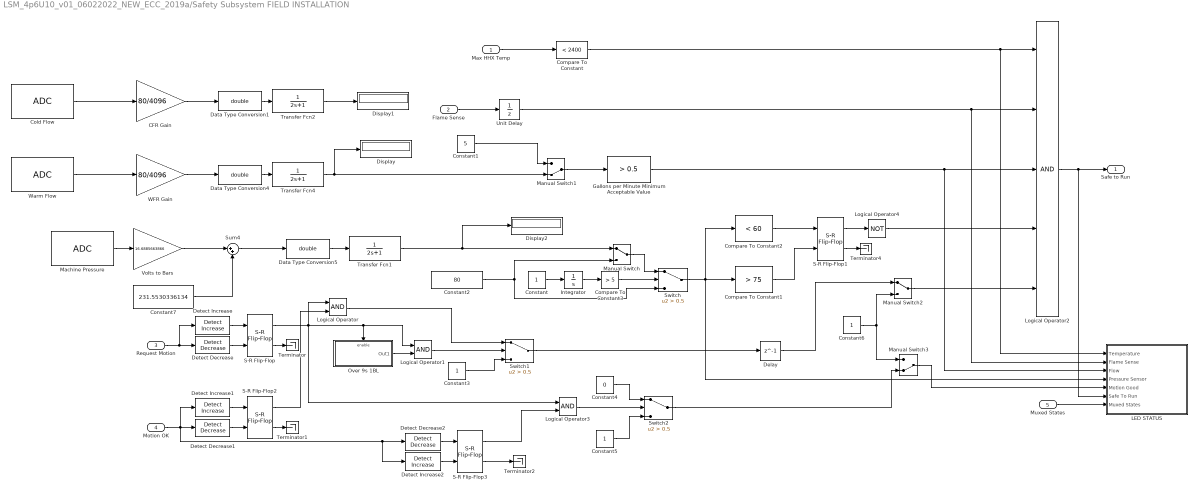
== system LSM_4p6U10_v01_06022022_NEW_ECC_2019a/Safety Subsystem FIELD INSTALLATION ==
  Max HHX Temp : Inport
  Flame Sense : Inport  Port=2
  Request Motion : Inport  Port=3
  Motion OK : Inport  Port=4
  Muxed States : Inport  Port=5
  CFR Gain : Gain  Gain=80/4096
  Cold Flow : c2802xlib/ADC  blkParamProc=C2000_Type4  ADCModule=A  samplingMode=Single sample mode  ADCResolution=12-bit (Single-ended input)  useSOC1=SOC11  useSOC2=SOC0_SOC1  SOCAcquisitionWindow=15  SOCTriggerSource=Software  SOCInterruptTrigger=No ADCINT  Ts=Ts_lowspeed  dType=uint16  postInterrupt=off  interruptSel=ADCINT1  ADCINTContinuous=on  endma=off  chdma=1  conv1=ADCINA0  conv2=ADCINA0 and ADCINB0  conv1_Type4=ADCIN5  conv2_Type4=ADCIN0 and ADCIN1
  Compare To Constant : simulink/Logic and Bit Operations/Compare To Constant  relop=<  const=2400  OutDataTypeStr=boolean
  Compare To Constant1 : simulink/Logic and Bit Operations/Compare To Constant  relop=>  const=75  OutDataTypeStr=boolean
  Compare To Constant2 : simulink/Logic and Bit Operations/Compare To Constant  relop=<  const=60  OutDataTypeStr=boolean
  Compare To Constant3 : simulink/Logic and Bit Operations/Compare To Constant  relop=>  const=5  OutDataTypeStr=boolean
  Constant : Constant
  Constant1 : Constant  Value=5
  Constant2 : Constant  Value=80  OutDataTypeStr=double
  Constant3 : Constant  OutDataTypeStr=boolean
  Constant4 : Constant  Value=0  OutDataTypeStr=boolean
  Constant5 : Constant  OutDataTypeStr=boolean
  Constant6 : Constant  OutDataTypeStr=boolean
  Constant7 : Constant  Value=231.5530336134
  Data Type Conversion1 : DataTypeConversion  OutDataTypeStr=double
  Data Type Conversion4 : DataTypeConversion  OutDataTypeStr=double
  Data Type Conversion5 : DataTypeConversion  OutDataTypeStr=double
  Delay : Delay  DelayLength=1
  Detect Decrease : simulink/Logic and Bit Operations/Detect Decrease  vinit=0.0  OutDataTypeStr=boolean
  Detect Decrease1 : simulink/Logic and Bit Operations/Detect Decrease  vinit=0.0  OutDataTypeStr=boolean
  Detect Decrease2 : simulink/Logic and Bit Operations/Detect Decrease  vinit=0.0  OutDataTypeStr=boolean
  Detect Increase : simulink/Logic and Bit Operations/Detect Increase  vinit=0.0  OutDataTypeStr=boolean
  Detect Increase1 : simulink/Logic and Bit Operations/Detect Increase  vinit=0.0  OutDataTypeStr=boolean
  Detect Increase2 : simulink/Logic and Bit Operations/Detect Increase  vinit=0.0  OutDataTypeStr=boolean
  Display : Display
  Display1 : Display
  Display2 : Display
  Gallons per Minute Minimum Acceptable Value : simulink/Logic and Bit Operations/Compare To Constant  relop=>  const=0.5  OutDataTypeStr=boolean
  Integrator : Integrator  LimitOutput=on  UpperSaturationLimit=6  LowerSaturationLimit=0
  LED STATUS : Subsystem
  Logical Operator : Logic  AllPortsSameDT=off  OutDataTypeStr=boolean
  Logical Operator1 : Logic  AllPortsSameDT=off  OutDataTypeStr=boolean
  Logical Operator2 : Logic  Inputs=5  AllPortsSameDT=off  OutDataTypeStr=boolean
  Logical Operator3 : Logic  AllPortsSameDT=off  OutDataTypeStr=boolean
  Logical Operator4 : Logic  Operator=NOT  AllPortsSameDT=off  OutDataTypeStr=boolean
  Machine Pressure : c2802xlib/ADC  blkParamProc=C2000_Type4  ADCModule=D  samplingMode=Single sample mode  ADCResolution=12-bit (Single-ended input)  useSOC1=SOC8  useSOC2=SOC0_SOC1  SOCAcquisitionWindow=15  SOCTriggerSource=Software  SOCInterruptTrigger=No ADCINT  Ts=Ts_lowspeed  dType=uint16  postInterrupt=off  interruptSel=ADCINT1  ADCINTContinuous=on  endma=off  chdma=1  conv1=ADCINA0  conv2=ADCINA0 and ADCINB0  conv1_Type4=ADCIN0  conv2_Type4=ADCIN0 and ADCIN1
  Manual Switch : ManualSwitch
  Manual Switch1 : ManualSwitch  CurrentSetting=0
  Manual Switch2 : ManualSwitch
  Manual Switch3 : ManualSwitch  CurrentSetting=0
  Over 9s 1BL : Subsystem
  S-R Flip-Flop{,1..3} (4 alike) : simulink_extras/Flip Flops/S-R Flip-Flop  initial_condition=0
  Sum4 : Sum  Inputs=|++
  Switch : Switch  Criteria=u2 > Threshold  Threshold=0.5
  Switch1 : Switch  Criteria=u2 > Threshold  Threshold=0.5
  Switch2 : Switch  Criteria=u2 > Threshold  Threshold=0.5
  Terminator{,1..2,4} (4 alike) : Terminator
  Transfer Fcn1 : TransferFcn  Denominator=[2 1]
  Transfer Fcn2 : TransferFcn  Denominator=[2 1]
  Transfer Fcn4 : TransferFcn  Denominator=[2 1]
  Unit Delay : UnitDelay  SampleTime=-1  HasFrameUpgradeWarning=on
  Volts to Bars : Gain  Gain=16.6885663866
  WFR Gain : Gain  Gain=80/4096
  Warm Flow : c2802xlib/ADC  blkParamProc=C2000_Type4  ADCModule=B  samplingMode=Single sample mode  ADCResolution=12-bit (Single-ended input)  useSOC1=SOC10  useSOC2=SOC0_SOC1  SOCAcquisitionWindow=15  SOCTriggerSource=Software  SOCInterruptTrigger=No ADCINT  Ts=Ts_lowspeed  dType=uint16  postInterrupt=off  interruptSel=ADCINT1  ADCINTContinuous=on  endma=off  chdma=1  conv1=ADCINA0  conv2=ADCINA0 and ADCINB0  conv1_Type4=ADCIN5  conv2_Type4=ADCIN0 and ADCIN1
  Safe to Run : Outport
  wires:
  Compare To Constant1/1 -> S-R Flip-Flop1/2
  S-R Flip-Flop1/1 -> Logical Operator4/1
  Logical Operator2/1 -> LED STATUS/6(Safe To Run), Safe to Run/1
  Constant2/1 -> Switch/3, Manual Switch/2
  Switch/1 -> LED STATUS/4(Pressure Sensor), Compare To Constant1/1, Compare To Constant2/1
  Transfer Fcn1/1 -> Display2/1, Manual Switch/1
  Data Type Conversion5/1 -> Transfer Fcn1/1
  Machine Pressure/1 -> Volts to Bars/1
  Data Type Conversion4/1 -> Transfer Fcn4/1
  Volts to Bars/1 -> Sum4/1
  S-R Flip-Flop1/2 -> Terminator4/1
  Warm Flow/1 -> WFR Gain/1
  Flame Sense/1 -> Unit Delay/1
  Logical Operator4/1 -> Logical Operator2/4
  Compare To Constant2/1 -> S-R Flip-Flop1/1
  Constant/1 -> Integrator/1
  Integrator/1 -> Compare To Constant3/1
  Compare To Constant3/1 -> Switch/2
  Manual Switch/1 -> Switch/1
  Transfer Fcn4/1 -> Display/1, Manual Switch1/2
  Constant1/1 -> Manual Switch1/1
  Manual Switch1/1 -> Gallons per Minute Minimum Acceptable Value/1
  Max HHX Temp/1 -> Compare To Constant/1
  Unit Delay/1 -> LED STATUS/2(Flame Sense), Logical Operator2/2
  Compare To Constant/1 -> Logical Operator2/1, LED STATUS/1(Temperature)
  Gallons per Minute Minimum Acceptable Value/1 -> LED STATUS/3(Flow), Logical Operator2/3
  Request Motion/1 -> Detect Increase/1, Detect Decrease/1
  Detect Increase/1 -> S-R Flip-Flop/1
  S-R Flip-Flop/1 -> Logical Operator1/1, Over 9s 1BL/Enable, Logical Operator3/1, Logical Operator/1
  S-R Flip-Flop/2 -> Terminator/1
  Detect Decrease/1 -> S-R Flip-Flop/2
  Switch1/1 -> Delay/1
  Detect Decrease1/1 -> S-R Flip-Flop2/2
  Detect Increase1/1 -> S-R Flip-Flop2/1
  S-R Flip-Flop2/1 -> Logical Operator/2
  S-R Flip-Flop2/2 -> Terminator1/1
  Motion OK/1 -> Detect Increase1/1, Detect Increase2/1, Detect Decrease2/1, Detect Decrease1/1
  Delay/1 -> Manual Switch2/1
  Constant3/1 -> Switch1/3
  Logical Operator1/1 -> Switch1/2
  Logical Operator/1 -> Switch1/1
  Over 9s 1BL/1(Out1) -> Logical Operator1/2
  Detect Increase2/1 -> S-R Flip-Flop3/2
  Detect Decrease2/1 -> S-R Flip-Flop3/1
  S-R Flip-Flop3/2 -> Terminator2/1
  S-R Flip-Flop3/1 -> Logical Operator3/2
  Logical Operator3/1 -> Switch2/2
  Constant4/1 -> Switch2/1
  Switch2/1 -> Manual Switch3/2
  Constant5/1 -> Switch2/3
  Constant6/1 -> Manual Switch3/1, Manual Switch2/2
  Manual Switch2/1 -> Logical Operator2/5
  Manual Switch3/1 -> LED STATUS/5(Motion Good)
  Muxed States/1 -> LED STATUS/7(Muxed States)
  Data Type Conversion1/1 -> Transfer Fcn2/1
  Cold Flow/1 -> CFR Gain/1
  Transfer Fcn2/1 -> Display1/1
  WFR Gain/1 -> Data Type Conversion4/1
  CFR Gain/1 -> Data Type Conversion1/1
  Constant7/1 -> Sum4/2
  Sum4/1 -> Data Type Conversion5/1

== system LSM_4p6U10_v01_06022022_NEW_ECC_2019a/Subsystem ==
  Enable : EnablePort  StatesWhenEnabling=reset
  Compare To Constant : simulink/Logic and Bit Operations/Compare To Constant  relop=<  const=2700  OutDataTypeStr=boolean
  Compare To Constant1 : simulink/Logic and Bit Operations/Compare To Constant  relop=>  const=3600  OutDataTypeStr=boolean
  Constant : Constant
  Delay : Delay  DelayLength=1
  Integrator : Integrator  ExternalReset=rising  LimitOutput=on  UpperSaturationLimit=3601  LowerSaturationLimit=0
  Out1 : Outport
  wires:
  Constant/1 -> Integrator/1
  Integrator/1 -> Compare To Constant1/1, Compare To Constant/1
  Compare To Constant/1 -> Out1/1
  Compare To Constant1/1 -> Delay/1
  Delay/1 -> Integrator/2

== system LSM_4p6U10_v01_06022022_NEW_ECC_2019a/System Initialize ==

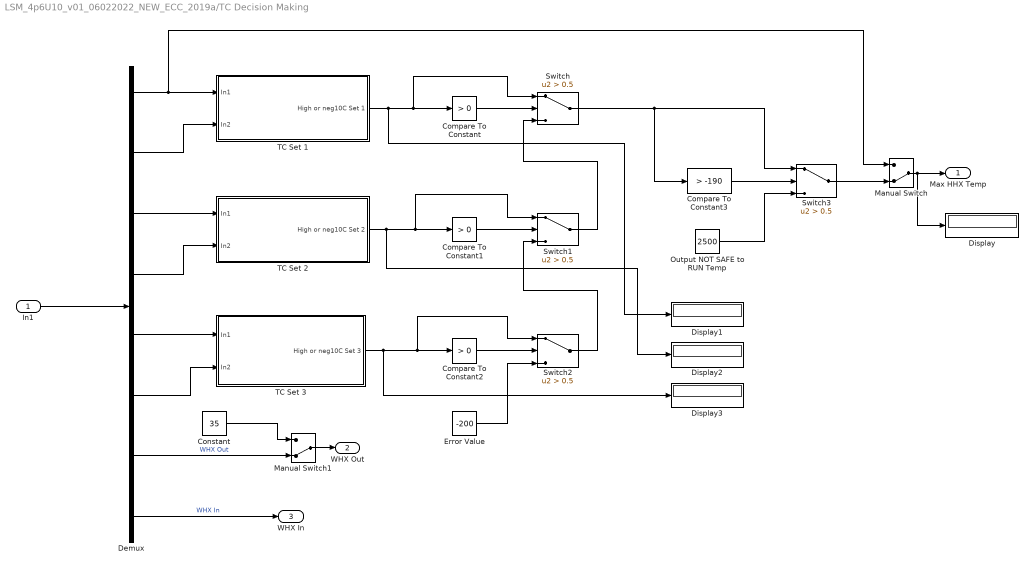
== system LSM_4p6U10_v01_06022022_NEW_ECC_2019a/TC Decision Making ==
  In1 : Inport
  Compare To Constant : simulink/Logic and Bit Operations/Compare To Constant  relop=>  const=0  OutDataTypeStr=boolean
  Compare To Constant1 : simulink/Logic and Bit Operations/Compare To Constant  relop=>  const=0  OutDataTypeStr=boolean
  Compare To Constant2 : simulink/Logic and Bit Operations/Compare To Constant  relop=>  const=0  OutDataTypeStr=boolean
  Compare To Constant3 : simulink/Logic and Bit Operations/Compare To Constant  relop=>  const=-190  OutDataTypeStr=boolean
  Constant : Constant  Value=35
  Demux : Demux  Outputs=8
  Display{,1..3} (4 alike) : Display
  Error Value : Constant  Value=-200
  Manual Switch : ManualSwitch  CurrentSetting=0
  Manual Switch1 : ManualSwitch  CurrentSetting=0
  Output NOT SAFE to RUN Temp : Constant  Value=2500
  Switch{,1..3} (4 alike) : Switch  Criteria=u2 > Threshold  Threshold=0.5
  TC Set 1 : Subsystem
  TC Set 2 : Subsystem
  TC Set 3 : Subsystem
  Max HHX Temp : Outport
  WHX Out : Outport  Port=2
  WHX In : Outport  Port=3
  wires:
  In1/1 -> Demux/1
  Demux/7 -> Manual Switch1/2  "WHX Out"
  Demux/8 -> WHX In/1  "WHX In"
  TC Set 1/1(High or neg10C Set 1) -> Display1/1, Switch/1, Compare To Constant/1
  TC Set 2/1(High or neg10C Set 2) -> Display2/1, Switch1/1, Compare To Constant1/1
  TC Set 3/1(High or neg10C Set 3) -> Display3/1, Switch2/1, Compare To Constant2/1
  Compare To Constant/1 -> Switch/2
  Compare To Constant1/1 -> Switch1/2
  Compare To Constant2/1 -> Switch2/2
  Switch/1 -> Switch3/1, Compare To Constant3/1
  Switch1/1 -> Switch/3
  Error Value/1 -> Switch2/3
  Switch2/1 -> Switch1/3
  Compare To Constant3/1 -> Switch3/2
  Output NOT SAFE to RUN Temp/1 -> Switch3/3
  Switch3/1 -> Manual Switch/2
  Manual Switch/1 -> Display/1, Max HHX Temp/1
  Manual Switch1/1 -> WHX Out/1
  Constant/1 -> Manual Switch1/1
  Demux/5 -> TC Set 3/1(In1)
  Demux/6 -> TC Set 3/2(In2)
  Demux/1 -> Manual Switch/1, TC Set 1/1(In1)
  Demux/2 -> TC Set 1/2(In2)
  Demux/3 -> TC Set 2/1(In1)
  Demux/4 -> TC Set 2/2(In2)

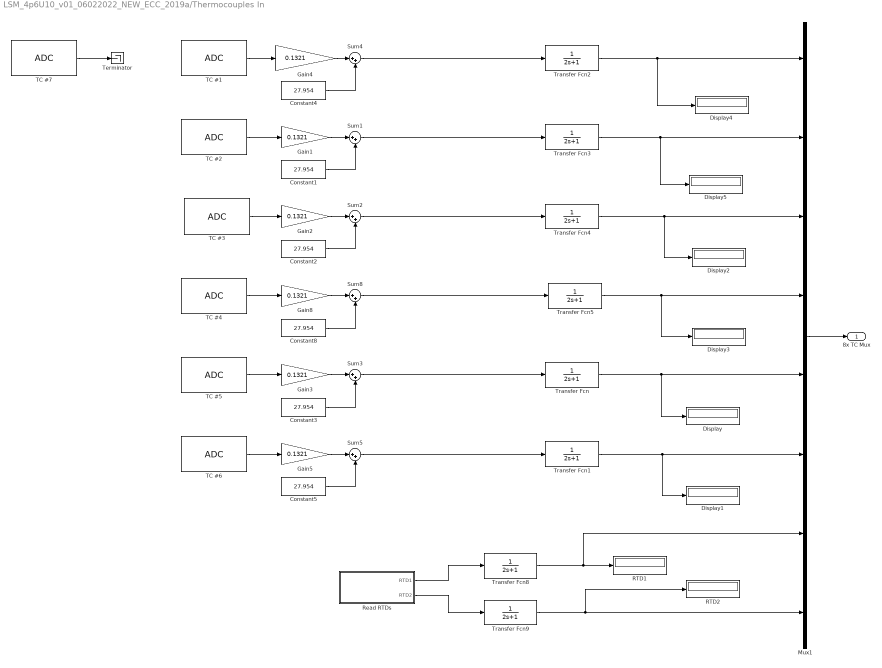
== system LSM_4p6U10_v01_06022022_NEW_ECC_2019a/Thermocouples In ==
  Constant{1..5,8} (6 alike) : Constant  Value=27.954
  Display{,1..5} (6 alike) : Display
  Gain{1..5,8} (6 alike) : Gain  Gain=0.1321
  Mux1 : Mux  Inputs=8
  RTD1 : Display
  RTD2 : Display
  Read RTDs : Subsystem
  Sum{1..5,8} (6 alike) : Sum  Inputs=|++
  TC #1 : c2802xlib/ADC  blkParamProc=C2000_Type4  ADCModule=C  samplingMode=Single sample mode  ADCResolution=12-bit (Single-ended input)  useSOC1=SOC0  useSOC2=SOC0_SOC1  SOCAcquisitionWindow=15  SOCTriggerSource=Software  SOCInterruptTrigger=No ADCINT  Ts=Ts_lowspeed  dType=uint16  postInterrupt=off  interruptSel=ADCINT1  ADCINTContinuous=on  endma=off  chdma=1  conv1=ADCINA0  conv2=ADCINA0 and ADCINB0  conv1_Type4=ADCIN3  conv2_Type4=ADCIN0 and ADCIN1
  TC #2 : c2802xlib/ADC  blkParamProc=C2000_Type4  ADCModule=B  samplingMode=Single sample mode  ADCResolution=12-bit (Single-ended input)  useSOC1=SOC1  useSOC2=SOC0_SOC1  SOCAcquisitionWindow=15  SOCTriggerSource=Software  SOCInterruptTrigger=No ADCINT  Ts=Ts_lowspeed  dType=uint16  postInterrupt=off  interruptSel=ADCINT1  ADCINTContinuous=on  endma=off  chdma=1  conv1=ADCINA0  conv2=ADCINA0 and ADCINB0  conv1_Type4=ADCIN3  conv2_Type4=ADCIN0 and ADCIN1
  TC #3 : c2802xlib/ADC  blkParamProc=C2000_Type4  ADCModule=A  samplingMode=Single sample mode  ADCResolution=12-bit (Single-ended input)  useSOC1=SOC2  useSOC2=SOC0_SOC1  SOCAcquisitionWindow=15  SOCTriggerSource=Software  SOCInterruptTrigger=No ADCINT  Ts=Ts_lowspeed  dType=uint16  postInterrupt=off  interruptSel=ADCINT1  ADCINTContinuous=on  endma=off  chdma=1  conv1=ADCINA0  conv2=ADCINA0 and ADCINB0  conv1_Type4=ADCIN3  conv2_Type4=ADCIN0 and ADCIN1
  TC #4 : c2802xlib/ADC  blkParamProc=C2000_Type4  ADCModule=C  samplingMode=Single sample mode  ADCResolution=12-bit (Single-ended input)  useSOC1=SOC3  useSOC2=SOC0_SOC1  SOCAcquisitionWindow=15  SOCTriggerSource=Software  SOCInterruptTrigger=No ADCINT  Ts=Ts_lowspeed  dType=uint16  postInterrupt=off  interruptSel=ADCINT1  ADCINTContinuous=on  endma=off  chdma=1  conv1=ADCINA0  conv2=ADCINA0 and ADCINB0  conv1_Type4=ADCIN2  conv2_Type4=ADCIN0 and ADCIN1
  TC #5 : c2802xlib/ADC  blkParamProc=C2000_Type4  ADCModule=B  samplingMode=Single sample mode  ADCResolution=12-bit (Single-ended input)  useSOC1=SOC4  useSOC2=SOC0_SOC1  SOCAcquisitionWindow=15  SOCTriggerSource=Software  SOCInterruptTrigger=No ADCINT  Ts=Ts_lowspeed  dType=uint16  postInterrupt=off  interruptSel=ADCINT1  ADCINTContinuous=on  endma=off  chdma=1  conv1=ADCINA0  conv2=ADCINA0 and ADCINB0  conv1_Type4=ADCIN2  conv2_Type4=ADCIN0 and ADCIN1
  TC #6 : c2802xlib/ADC  blkParamProc=C2000_Type4  ADCModule=A  samplingMode=Single sample mode  ADCResolution=12-bit (Single-ended input)  useSOC1=SOC5  useSOC2=SOC0_SOC1  SOCAcquisitionWindow=15  SOCTriggerSource=Software  SOCInterruptTrigger=No ADCINT  Ts=Ts_lowspeed  dType=uint16  postInterrupt=off  interruptSel=ADCINT1  ADCINTContinuous=on  endma=off  chdma=1  conv1=ADCINA0  conv2=ADCINA0 and ADCINB0  conv1_Type4=ADCIN2  conv2_Type4=ADCIN0 and ADCIN1
  TC #7 : c2802xlib/ADC  blkParamProc=C2000_Type4  ADCModule=A  samplingMode=Single sample mode  ADCResolution=12-bit (Single-ended input)  useSOC1=SOC6  useSOC2=SOC0_SOC1  SOCAcquisitionWindow=15  SOCTriggerSource=Software  SOCInterruptTrigger=No ADCINT  Ts=0.1  dType=uint16  postInterrupt=off  interruptSel=ADCINT1  ADCINTContinuous=on  endma=off  chdma=1  conv1=ADCINA0  conv2=ADCINA0 and ADCINB0  conv1_Type4=ADCIN0  conv2_Type4=ADCIN0 and ADCIN1
  Terminator : Terminator
  Transfer Fcn{,1..5,8..9} (8 alike) : TransferFcn  Denominator=[2 1]
  8x TC Mux : Outport
  wires:
  Sum3/1 -> Transfer Fcn/1
  Transfer Fcn/1 -> Mux1/5, Display/1
  Mux1/1 -> 8x TC Mux/1
  Sum5/1 -> Transfer Fcn1/1
  Sum2/1 -> Transfer Fcn4/1
  Sum8/1 -> Transfer Fcn5/1
  Sum1/1 -> Transfer Fcn3/1
  Constant4/1 -> Sum4/2
  Sum4/1 -> Transfer Fcn2/1
  Transfer Fcn1/1 -> Mux1/6, Display1/1
  Transfer Fcn4/1 -> Display2/1, Mux1/3
  Transfer Fcn5/1 -> Mux1/4, Display3/1
  Transfer Fcn2/1 -> Mux1/1, Display4/1
  Transfer Fcn3/1 -> Mux1/2, Display5/1
  Gain4/1 -> Sum4/1
  Gain1/1 -> Sum1/1
  Constant1/1 -> Sum1/2
  Constant2/1 -> Sum2/2
  Gain2/1 -> Sum2/1
  Gain5/1 -> Sum5/1
  Constant5/1 -> Sum5/2
  Constant3/1 -> Sum3/2
  Gain3/1 -> Sum3/1
  Gain8/1 -> Sum8/1
  Constant8/1 -> Sum8/2
  TC #2/1 -> Gain1/1
  TC #1/1 -> Gain4/1
  TC #4/1 -> Gain8/1
  TC #3/1 -> Gain2/1
  TC #5/1 -> Gain3/1
  TC #6/1 -> Gain5/1
  TC #7/1 -> Terminator/1
  Transfer Fcn8/1 -> Mux1/7, RTD1/1
  Transfer Fcn9/1 -> RTD2/1, Mux1/8
  Read RTDs/1(RTD1) -> Transfer Fcn8/1
  Read RTDs/2(RTD2) -> Transfer Fcn9/1
